simulink model "Inciso_C_Simulink"  (R2024b)
settings: Solver=ode45  StartTime=0.0  StopTime=10  RelTol=1e-3
undefined symbols (not defined in the file or in its folder): Kd, Kp
settings Model: Creator=Lenovo  LastModifiedBy=Lenovo

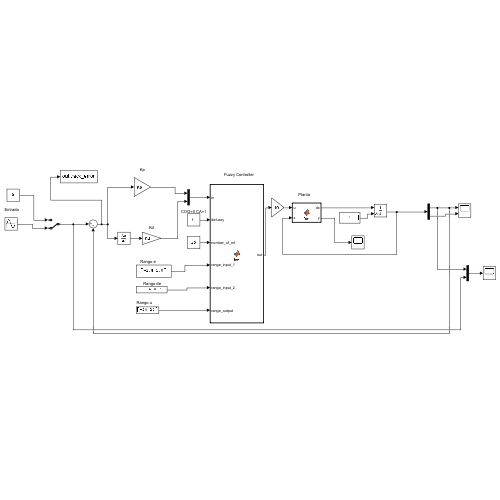
[thumbnail: Simulink's stored preview of the top-level diagram]
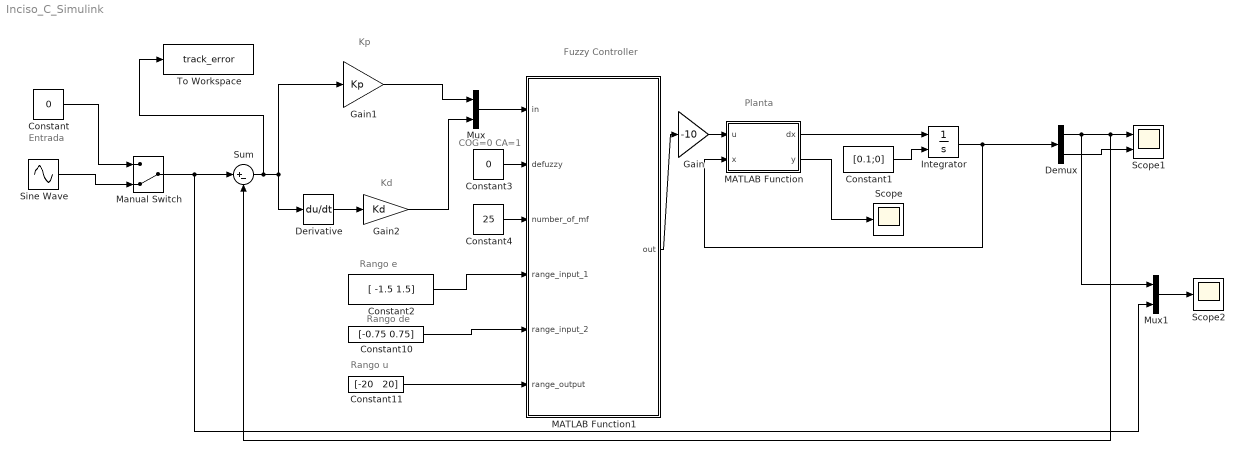
== system Inciso_C_Simulink ==
  note: COG=0 CA=1
  note: Rango u
  note: Rango de
  note: Rango e
  note: Entrada
  note: Kd
  note: Kp
  note: Planta
  note: Fuzzy Controller
  Constant : Constant  Value=0
  Constant1 : Constant  Value=[0.1;0]
  Constant10 : Constant  Value=[-0.75 0.75]
  Constant11 : Constant  Value="[-20   20]"
  Constant2 : Constant  Value=[ -1.5 1.5]
  Constant3 : Constant  Value=0
  Constant4 : Constant  Value=25
  Demux : Demux  Outputs=2
  Derivative : Derivative
  Gain : Gain  Gain=-10
  Gain1 : Gain  Gain=Kp
  Gain2 : Gain  Gain=Kd
  Integrator : Integrator  InitialConditionSource=external
  MATLAB Function : MATLAB Function  TreatAsAtomicUnit=on
  MATLAB Function1 : MATLAB Function  TreatAsAtomicUnit=on
  Manual Switch : ManualSwitch  CurrentSetting=0
  Mux : Mux  Inputs=2
  Mux1 : Mux  Inputs=2
  Scope : Scope
  Scope1 : Scope  NumInputPorts=2
  Scope2 : Scope
  Sine Wave : Sin  Amplitude=.25  Frequency=4  SampleTime=0
  Sum : Sum  Inputs=|+-
  To Workspace : ToWorkspace  VariableName=track_error  SampleTime=-1
  wires:
  Integrator/1 -> Demux/1, MATLAB Function/2(x)
  MATLAB Function/1(dx) -> Integrator/1
  Constant1/1 -> Integrator/2
  Demux/1 -> Mux1/1, Sum/2, Scope1/1
  Demux/2 -> Scope1/2
  MATLAB Function/2(y) -> Scope/1
  Gain/1 -> MATLAB Function/1(u)
  MATLAB Function1/1(out) -> Gain/1
  Gain1/1 -> Mux/1
  Derivative/1 -> Gain2/1
  Sum/1 -> To Workspace/1, Derivative/1, Gain1/1
  Manual Switch/1 -> Mux1/2, Sum/1
  Constant/1 -> Manual Switch/1
  Sine Wave/1 -> Manual Switch/2
  Mux1/1 -> Scope2/1
  Constant4/1 -> MATLAB Function1/3(number_of_mf)
  Constant2/1 -> MATLAB Function1/4(range_input_1)
  Constant10/1 -> MATLAB Function1/5(range_input_2)
  Constant11/1 -> MATLAB Function1/6(range_output)
  Gain2/1 -> Mux/2
  Mux/1 -> MATLAB Function1/1(in)
  Constant3/1 -> MATLAB Function1/2(defuzzy)

== matlab function Inciso_C_Simulink/MATLAB Function1 ==
  data: in input; out output; defuzzy input; number_of_mf input; range_input_1 input; range_input_2 input; range_output input
function out = fcn(in, defuzzy, number_of_mf, range_input_1, range_input_2, range_output)
% in: [error, d_error]
% defuzzy: 0 = COG, 1 = CA
% range_input_1/2: [min, max]
% range_output: [min, max]

% === 1. Divisiones (uniformes, como linspace) ===
n = number_of_mf;
div1    = linspace(range_input_1(1), range_input_1(2), n);  % error
div2    = linspace(range_input_2(1), range_input_2(2), n);  % d_error
div_out = linspace(range_output(1),  range_output(2),  n);  % salida

% === 2. Membresías triangulares uniformes ===
mu_e  = compute_memberships(in(1), div1);
mu_de = compute_memberships(in(2), div2);

% === 3. FAM PD simétrica (con redondeo de etiqueta) ===
FAM = zeros(n,n);
c   = (n + 1)/2;                  % puede ser .5 si n es par
for i = 1:n
    for j = 1:n
        v = c + (2*c) - (i + j);  % 3c - (i+j)
        v = round(v);             % <-- CORRECCIÓN: etiqueta entera
        if v < 1, v = 1; elseif v > n, v = n; end
        FAM(i,j) = v;
    end
end

% === 4. Activaciones (min) y agregación por etiqueta (max) ===
rule_heights = zeros(n,n);
for i = 1:n
    for j = 1:n
        rule_heights(i,j) = min(mu_e(i), mu_de(j));
    end
end

mu_out = zeros(1,n);
for k = 1:n
    mask = (FAM == k);                 % reglas que salen con etiqueta k
    if any(mask(:))                    % evita max([]) cuando n es par
        mu_out(k) = max(rule_heights(mask));
    else
        mu_out(k) = 0;
    end
end

% === 5. Defuzzificación ===
% Centro robusto (sirve para n impar/par)
midL = floor((n+1)/2);
midR = ceil((n+1)/2);
center_val = 0.5*(div_out(midL) + div_out(midR));

if defuzzy == 0
    % --- COG (centroide) con trapecios truncados ---
    num = 0; den = 0;
    if n >= 2
        step = div_out(2) - div_out(1);
    else
        step = 0;
    end
    base = 2*step;         % base total del triángulo
    for k = 1:n
        h = mu_out(k);
        if h > 0
            top_base = (1-h)*base;
            A = h*(base + top_base)/2; % área del trapecio truncado
            num = num + A*div_out(k);
            den = den + A;
        end
    end
    if den == 0
        out = center_val;
    else
        out = num/den;
    end
else
    % --- CA (promedio ponderado por alturas) ---
    num = sum(mu_out .* div_out);
    den = sum(mu_out);
    if den == 0
        out = center_val;
    else
        out = num/den;
    end
end
end

% === Membresías triangulares uniformes ===
function mu = compute_memberships(x, div)
n = length(div);
mu = zeros(1,n);

if x <= div(1)
    mu(1) = 1; 
    return
elseif x >= div(end)
    mu(end) = 1; 
    return
end

for i = 1:n-1
    x1 = div(i); x2 = div(i+1);
    if x >= x1 && x <= x2
        den = x2 - x1; if den == 0, den = eps; end
        mu(i)   = (x2 - x)/den;
        mu(i+1) = (x  - x1)/den;
        return
    end
end
% si no cae en ningún intervalo (redondeos), queda en ceros
end

== matlab function Inciso_C_Simulink/MATLAB Function ==
  data: dx output; u input; y output; x input
function [dx, y] = fcn(u,x)

k=2;
b=0.2;
m=1;
x1=x(1);
x2=x(2);
dx1=x2;
dx2=b*x2/m-k*x1/m+u/m;
dx = [dx1;dx2];

y = x1;
